simulink model "relay_with_flipflop"  (R2025b)
settings: Solver=VariableStepAuto  StartTime=0.0  StopTime=10.0  RelTol=1e-3
libraries: simulink x2, simulink_extras x1
settings Model: Creator=daniel  LastModifiedBy=daniel

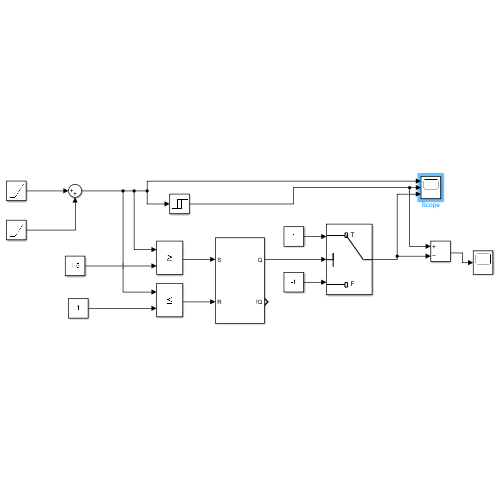
[thumbnail: Simulink's stored preview of the top-level diagram]
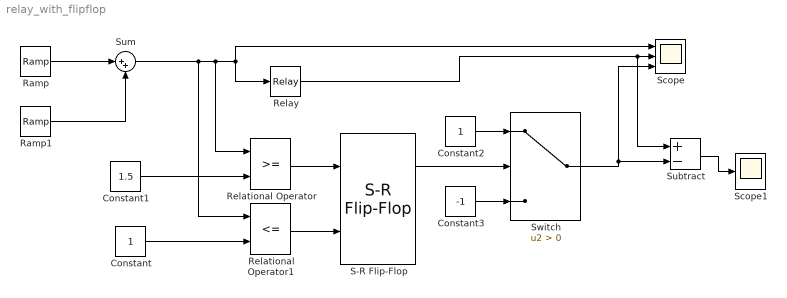
== system relay_with_flipflop ==
  Constant : Constant
  Constant1 : Constant  Value=1.5
  Constant2 : Constant
  Constant3 : Constant  Value=-1
  Ramp : simulink/Sources/Ramp  slope=1  start=0  InitialOutput=0
  Ramp1 : simulink/Sources/Ramp  slope=-2  start=3  InitialOutput=0
  Relational Operator : RelationalOperator  OutDataTypeStr=boolean  RndMeth=Simplest  InputSameDT=off
  Relational Operator1 : RelationalOperator  Operator=<=  OutDataTypeStr=boolean  RndMeth=Simplest  InputSameDT=off
  Relay : Relay  OnSwitchValue=1.5  OffSwitchValue=1  OffOutputValue=-1
  S-R Flip-Flop : simulink_extras/Flip Flops/S-R Flip-Flop  initial_condition=0
  Scope : Scope  NumInputPorts=3
      settings: ActiveDisplayYMinimum=-2.0281157032276673  ActiveDisplayYMaximum=3.3743122657106688
  Scope1 : Scope
      settings: ActiveDisplayYMinimum=-1.8787968946104956  ActiveDisplayYMaximum=1.1802660562699137
  Subtract : Sum  Inputs=+-
  Sum : Sum  Inputs=|++
  Switch : Switch  Criteria=u2 > Threshold  SaturateOnIntegerOverflow=off  InputSameDT=off
  wires:
  Ramp/1 -> Sum/1
  Relay/1 -> Subtract/1, Scope/2
  Ramp1/1 -> Sum/2
  Sum/1 -> Relational Operator1/1, Relational Operator/1, Relay/1, Scope/1
  Constant1/1 -> Relational Operator/2
  Constant/1 -> Relational Operator1/2
  Relational Operator/1 -> S-R Flip-Flop/1
  Relational Operator1/1 -> S-R Flip-Flop/2
  S-R Flip-Flop/1 -> Switch/2
  Constant2/1 -> Switch/1
  Constant3/1 -> Switch/3
  Switch/1 -> Subtract/2, Scope/3
  Subtract/1 -> Scope1/1
